simulink model "Execution_servo_tangage_4_tempo_v2"  (R2018a)
settings: Solver=FixedStepDiscrete  StartTime=0.0  StopTime=inf  RelTol=1e-3  EnableMultiTasking=on
libraries: arduinolib x3, realtime_pacer_lib x1
settings Model: SimulationMode=external  ExtModeTrigDuration=2  Creator=Francois  LastModifiedBy=admin-local
settings DataIOCC: LimitDataPoints=on  SaveFormat=Array  SignalLoggingSaveFormat=ModelDataLogs
settings OptimizationCC: EnhancedBackFolding=on  PassReuseOutputArgsAs=Individual arguments  ExpressionDepthLimit=2147483647  MaxStackSize=64  OptimizeBlockOrder=speed  DifferentSizesBufferReuse=on  OptimizationCustomize=off
settings DebuggingCC: UnderspecifiedInitializationDetection=Classic  MergeDetectMultiDrivingBlocksExec=none  SolverPrmCheckMsg=warning  ParameterTunabilityLossMsg=error  FcnCallInpInsideContextMsg=warning  StateNameClashWarn=warning  SFUnexpectedBacktrackingDiag=warning  SFNoUnconditionalDefaultTransitionDiag=warning  SFExecutionAtInitializationDiag=none
settings HardwareCC: ProdBitPerInt=16  ProdBitPerPointer=16  ProdBitPerSizeT=16  ProdBitPerPtrDiffT=16  ProdLargestAtomicFloat=None  ProdWordSize=8  ProdHWDeviceType=Atmel->AVR
settings ModelReferenceCC: PropagateSignalLabelsOutOfModel=off
settings SFSimCC: MATLABDynamicMemAlloc=off
settings RTWCC: SystemTargetFile=ert.tlc  HardwareBoard=Arduino Uno  TLCOptions=-aInlineSetEventsForThisBaseRateFcn=TLC_FALSE -aSuppressMultiTaskScheduler=TLC_FALSE -aRateBasedStepFcn=1  TemplateMakefile=ert_default_tmf  GenerateReport=on  Toolchain=Arduino AVR  BuildConfiguration=Faster Runs  IncludeHyperlinkInReport=on  LaunchReport=on  GenerateTraceInfo=on  GenerateTraceReport=on  GenerateTraceReportSl=on  GenerateTraceReportSf=on  GenerateTraceReportEml=on
settings CodeAppCC: ForceParamTrailComments=on  IgnoreCustomStorageClasses=off  OperatorAnnotations=on  SimulinkDataObjDesc=on  SFDataObjDesc=on  InsertBlockDesc=on
settings ERTTargetCC: SupportContinuousTime=on  SupportVariableSizeSignals=on
settings ConfigComp: CovMetricSettings=dw  CovHtmlReporting=on  CovSaveCumulativeToWorkspaceVar=on  CovSaveSingleToWorkspaceVar=on  CovExternalEMLEnable=off

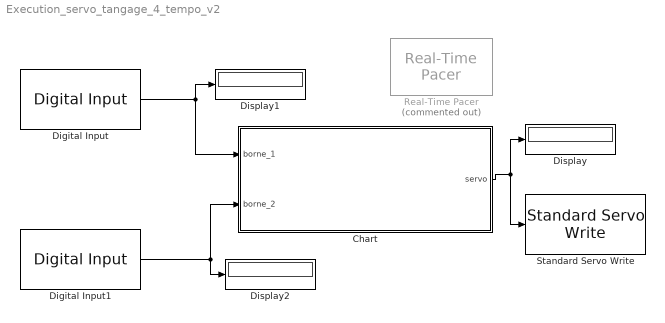
== system Execution_servo_tangage_4_tempo_v2 ==
  Chart : Stateflow chart  TreatAsAtomicUnit=on
  Digital Input : arduinolib/Digital Input  pinNumber=2  sampleTime=0.1  blockPlatform=arduino
      settings: SourceProductName=Simulink Support Package for Arduino Hardware
  Digital Input1 : arduinolib/Digital Input  pinNumber=4  sampleTime=0.1  blockPlatform=arduino
      settings: SourceProductName=Simulink Support Package for Arduino Hardware
  Display : Display
  Display1 : Display
  Display2 : Display
  Real-Time Pacer : realtime_pacer_lib/Real-Time Pacer  Commented=on  simTimePerRealTime=1
  Standard Servo Write : arduinolib/Standard Servo Write  pinNumber=3  blockPlatform=arduino
      settings: SourceProductName=Simulink Support Package for Arduino Hardware
  wires:
  Digital Input/1 -> Chart/1(borne_1), Display1/1
  Digital Input1/1 -> Chart/2(borne_2), Display2/1
  Chart/1(servo) -> Standard Servo Write/1, Display/1

== stateflow chart Execution_servo_tangage_4_tempo_v2/Chart ==
  state init
  state tangage_libre
    during : servo = 130;
  state tangage_limite
    during : servo = 90;
  state tangage_bloque
    during : servo = 50;
  state mvt_controle
    state rapide
      entry : servo = 60;
    state incremente
      entry : servo = servo -1;
    (default) -> rapide
    incremente -> (junction 31) : after(0.1,sec)
    (junction 31) -> incremente : [servo>50]
    rapide -> incremente : [servo>50]
  init -> tangage_libre [order 1] : [borne_1 && !borne_2]
  (default) -> init
  tangage_limite -> tangage_libre [order 2] : [borne_1 && !borne_2]
  tangage_libre -> tangage_limite : [! borne_1]
  init -> tangage_limite [order 3] : [borne_1 == 0 && borne_2 == 1]
  init -> mvt_controle [order 2] : [borne_1==1 && borne_2==1]
  tangage_limite -> mvt_controle [order 1] : [borne_1 == 1 && borne_2 == 1]
  tangage_bloque -> tangage_limite : [borne_1 == 0 && borne_2 == 1]
  mvt_controle -> tangage_bloque : [servo == 50]
  data: borne_1 input; borne_2 input; servo output double
